simulink library "sun_sensor_lib"  (R2016b)
settings: Solver=VariableStepAuto  StartTime=0.0  StopTime=10.0  RelTol=1e-3
undefined symbols (not defined in the file or in its folder): magnitude
libraries: aerolibutil x1, aerolibtransform2 x1
settings Model: Creator=Taylor  LastModifiedBy=Taylor
settings OptimizationCC: LifeSpan=inf
settings DebuggingCC: SFExecutionAtInitializationDiag=none

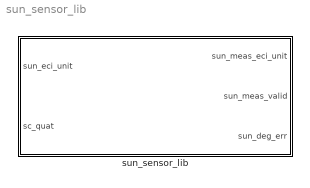
== system sun_sensor_lib ==
  "sun_sensor_lib " : Subsystem

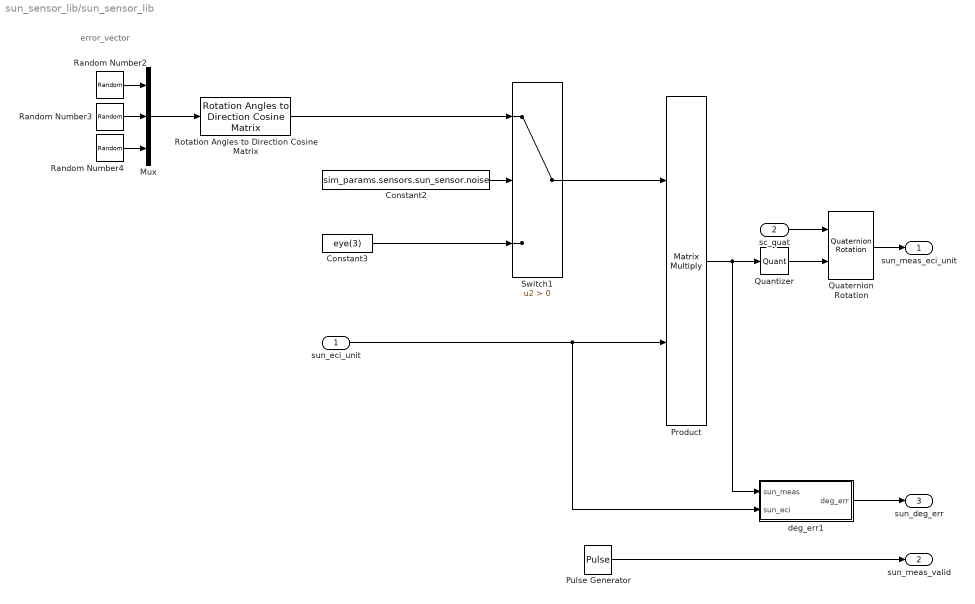
== system sun_sensor_lib/sun_sensor_lib  ==
  note: error_vector
  sun_eci_unit : Inport
  sc_quat : Inport  Port=2
  Constant2 : Constant  Value=sim_params.sensors.sun_sensor.noise
  Constant3 : Constant  Value=eye(3)
  Mux : Mux  Inputs=3
  Product : Product  Multiplication=Matrix(*)  RndMeth=Zero
  Pulse Generator : DiscretePulseGenerator  PulseType=Time based  Period=10  PulseWidth=sim_params.sensors.sun_sensor.valid_pct
  Quantizer : Quantizer  QuantizationInterval=sim_params.sensors.sun_sensor.resolution
  Quaternion Rotation : aerolibutil/Quaternion Rotation
  Random Number2 : RandomNumber  Variance=sim_params.sensors.sun_sensor.varx  SampleTime=sim_params.sensors.sun_sensor.sample_time_s
  Random Number3 : RandomNumber  Variance=sim_params.sensors.sun_sensor.vary  Seed=1  SampleTime=sim_params.sensors.sun_sensor.sample_time_s
  Random Number4 : RandomNumber  Variance=sim_params.sensors.sun_sensor.varz  Seed=2  SampleTime=sim_params.sensors.sun_sensor.sample_time_s
  Rotation Angles to Direction Cosine Matrix : aerolibtransform2/Rotation Angles to Direction Cosine Matrix  rotationOrder=ZYX
  Switch1 : Switch  Criteria=u2 > Threshold
  deg_err1 : Subsystem
  sun_meas_eci_unit : Outport
  sun_meas_valid : Outport  Port=2
  sun_deg_err : Outport  Port=3
  wires:
  Quaternion Rotation/1 -> sun_meas_eci_unit/1
  sc_quat/1 -> Quaternion Rotation/1
  Pulse Generator/1 -> sun_meas_valid/1
  Constant2/1 -> Switch1/2
  Constant3/1 -> Switch1/3
  Switch1/1 -> Product/1
  sun_eci_unit/1 -> deg_err1/2(sun_eci), Product/2
  Rotation Angles to Direction Cosine Matrix/1 -> Switch1/1
  Product/1 -> deg_err1/1(sun_meas), Quantizer/1
  Quantizer/1 -> Quaternion Rotation/2
  Mux/1 -> Rotation Angles to Direction Cosine Matrix/1
  Random Number3/1 -> Mux/2
  Random Number2/1 -> Mux/1
  Random Number4/1 -> Mux/3
  deg_err1/1(deg_err) -> sun_deg_err/1

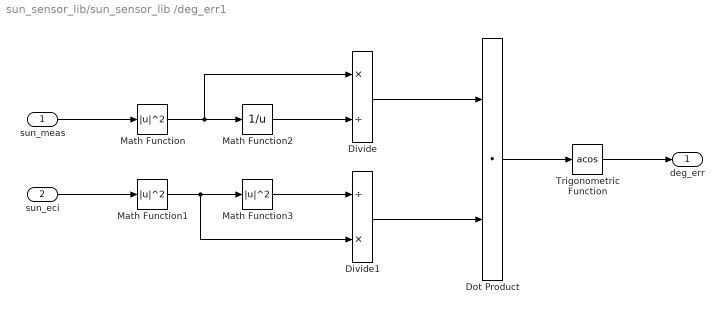
== system sun_sensor_lib/sun_sensor_lib /deg_err1 ==
  sun_meas : Inport
  sun_eci : Inport  Port=2
  Divide : Product  Inputs=*/
  Divide1 : Product  Inputs=/*
  Dot Product : DotProduct  InputSameDT=on  OutDataTypeStr=Inherit: Inherit via internal rule
  Math Function : Math  Operator=magnitude^2  SaturateOnIntegerOverflow=on
  Math Function1 : Math  Operator=magnitude^2  SaturateOnIntegerOverflow=on
  Math Function2 : Math  Operator=reciprocal  SaturateOnIntegerOverflow=on
  Math Function3 : Math  Operator=magnitude^2  SaturateOnIntegerOverflow=on
  Trigonometric Function : Trigonometry  Operator=acos
  deg_err : Outport
  wires:
  Trigonometric Function/1 -> deg_err/1
  Dot Product/1 -> Trigonometric Function/1
  Divide1/1 -> Dot Product/2
  Math Function1/1 -> Math Function3/1, Divide1/2
  Math Function3/1 -> Divide1/1
  sun_eci/1 -> Math Function1/1
  Divide/1 -> Dot Product/1
  Math Function2/1 -> Divide/2
  Math Function/1 -> Math Function2/1, Divide/1
  sun_meas/1 -> Math Function/1
